simulink model "sampleModel1862"  (R2023a)
settings: Solver=VariableStepAuto  StartTime=0.0  StopTime=10.0  RelTol=1e-3
libraries: hdlsllib x1, simulink x1
settings Model: Creator=user1  LastModifiedBy=user1

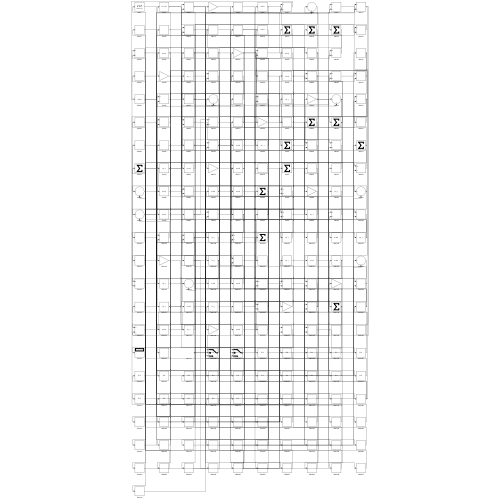
[thumbnail: Simulink's stored preview of the top-level diagram]
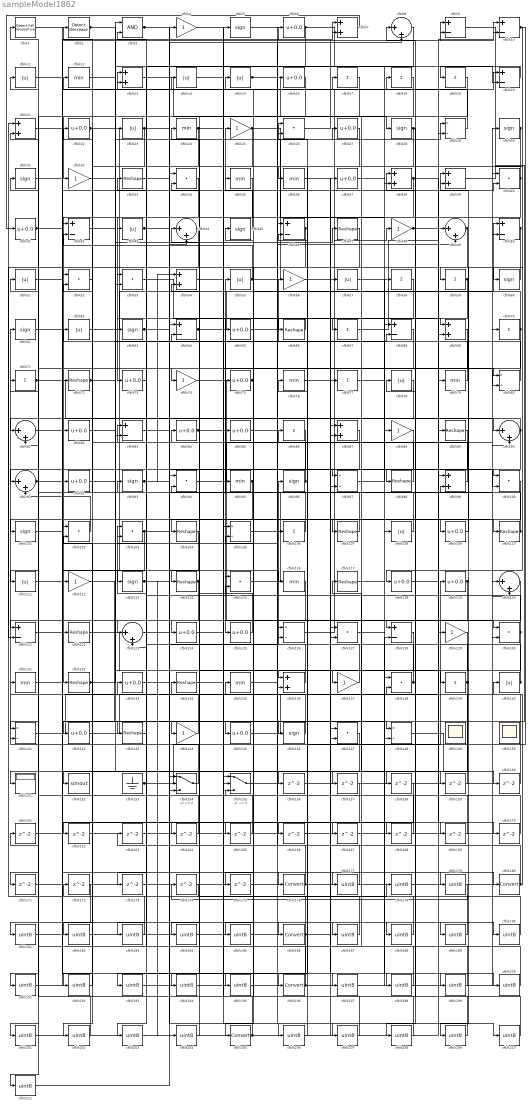
== system sampleModel1862 ==
  cfblk1 : hdlsllib/Logic and Bit Operations/Detect Fall Nonpositive  vinit=0  OutDataTypeStr=boolean
  cfblk{9..10,20,42,46,50,64,68,83,121,128} (11 alike) : Sum  Inputs=+-
  cfblk{26,34,40,52..53,94,100,102..103,115,127,130,138,147} (14 alike) : DotProduct  OutDataTypeStr=Inherit: Inherit via internal rule
  cfblk{5,28,30..31,45,60..61,63,93,96,101,113,146} (13 alike) : Signum
  cfblk{33,47,66,72,89,98,104,107,110,114,117,122,132,134,143} (15 alike) : Reshape
  cfblk{29,80,97,105,126,141,148} (7 alike) : Product  Inputs=*/  RndMeth=Zero  SaturateOnIntegerOverflow=on
  cfblk{17..19,58..59,67,70..71,77,86,106,139} (12 alike) : Sum  Inputs=+
  cfblk{11,14..15,23,43,51,55,57,62,78,108,111,140} (13 alike) : Abs  SaturateOnIntegerOverflow=off
  cfblk{6,16,22,27,37,41,65,73,75,82,84..85,92,109,118..119,124..125,133,142,145} (21 alike) : Bias  Bias=0.0  SaturateOnIntegerOverflow=off
  cfblk{4,25,32,48,56,74,88,112,129,137,144} (11 alike) : Gain
  cfblk{12,24,35..36,76,79,95,116,131,135} (10 alike) : MinMax
  cfblk{8,44,49,81,90..91,120,123} (8 alike) : Sum  Inputs=|++
  cfblk{7,13,21,38..39,54,69,87,99,136} (10 alike) : Sum
  cfblk149 : Scope
      settings: Floating=on
  cfblk150 : Scope
      settings: Floating=on
  cfblk151 : Display
  cfblk152 : ToWorkspace  VariableName=simout  SaveFormat=Timeseries  SampleTime=-1
  cfblk153 : Ground
  cfblk154 : Switch  SaturateOnIntegerOverflow=off  InputSameDT=off
  cfblk155 : Switch  SaturateOnIntegerOverflow=off  InputSameDT=off
  cfblk{156..175} (20 alike) : Delay  SampleTime=1
  cfblk{176,180,186,196,205} (5 alike) : DataTypeConversion  SaturateOnIntegerOverflow=off  RndMeth=Floor
  cfblk{177..179,181..185,187..195,197..204,206..211} (31 alike) : DataTypeConversion  OutDataTypeStr=uint8  SaturateOnIntegerOverflow=off  RndMeth=Floor
  cfblk2 : simulink/Logic and Bit Operations/Detect Decrease  vinit=0.0  OutDataTypeStr=boolean
      settings: LibrarySourceBlock=|
      | hdlsllib/Logic and Bit
      | Operations/Detect
      | Decrease
  cfblk3 : Logic  AllPortsSameDT=off  OutDataTypeStr=boolean
  wires:
  cfblk99/1 -> cfblk55/1
  cfblk44/1 -> cfblk132/1
  cfblk33/1 -> cfblk176/1
  cfblk113/1 -> cfblk204/1, cfblk206/1
  cfblk56/1 -> cfblk18/1
  cfblk22/1 -> cfblk114/1, cfblk82/1
  cfblk109/1 -> cfblk13/1
  cfblk38/1 -> cfblk73/1, cfblk170/1
  cfblk40/1 -> cfblk92/1, cfblk36/1
  cfblk55/1 -> cfblk29/1, cfblk42/2
  cfblk64/1 -> cfblk50/1, cfblk80/2
  cfblk85/1 -> cfblk130/1
  cfblk140/1 -> cfblk103/1, cfblk115/2
  cfblk46/1 -> cfblk104/1, cfblk65/1
  cfblk39/1 -> cfblk118/1
  cfblk126/1 -> cfblk48/1
  cfblk71/1 -> cfblk90/1, cfblk113/1
  cfblk60/1 -> cfblk59/1
  cfblk6/1 -> cfblk53/1, cfblk38/2
  cfblk154/1 -> cfblk61/1
  cfblk110/1 -> cfblk12/1, cfblk26/1
  cfblk96/1 -> cfblk91/1, cfblk52/2
  cfblk50/1 -> cfblk74/1, cfblk109/1
  cfblk112/1 -> cfblk144/1
  cfblk129/1 -> cfblk196/1
  cfblk70/1 -> cfblk39/2, cfblk181/1
  cfblk15/1 -> cfblk28/1, cfblk187/1
  cfblk63/1 -> cfblk9/1, cfblk87/2
  cfblk17/1 -> cfblk124/1
  cfblk80/1 -> cfblk56/1
  cfblk146/1 -> cfblk134/1
  cfblk9/1 -> cfblk148/1
  cfblk88/1 -> cfblk111/1
  cfblk62/1 -> cfblk16/1
  cfblk10/1 -> cfblk136/1, cfblk60/1
  cfblk108/1 -> cfblk15/1
  cfblk35/1 -> cfblk43/1
  cfblk20/1 -> cfblk19/1
  cfblk18/1 -> cfblk32/1
  cfblk45/1 -> cfblk25/1
  cfblk122/1 -> cfblk136/2
  cfblk91/1 -> cfblk148/2, cfblk159/1
  cfblk7/1 -> cfblk41/1
  cfblk145/1 -> cfblk89/1
  cfblk86/1 -> cfblk205/1
  cfblk29/1 -> cfblk2/1
  cfblk68/1 -> cfblk152/1
  cfblk74/1 -> cfblk128/1
  cfblk143/1 -> cfblk93/1
  cfblk98/1 -> cfblk24/1
  cfblk58/1 -> cfblk66/1
  cfblk138/1 -> cfblk83/1, cfblk38/1
  cfblk153/1 -> cfblk119/1, cfblk126/2
  cfblk84/1 -> cfblk64/2, cfblk20/1
  cfblk141/1 -> cfblk133/1
  cfblk144/1 -> cfblk11/1
  cfblk48/1 -> cfblk49/1, cfblk100/2
  cfblk82/1 -> cfblk3/1
  cfblk92/1 -> cfblk23/1
  cfblk53/1 -> cfblk69/1
  cfblk155/1 -> cfblk46/1
  cfblk135/1 -> cfblk49/2
  cfblk52/1 -> cfblk22/1
  cfblk87/1 -> cfblk151/1
  cfblk59/1 -> cfblk125/1, cfblk39/1
  cfblk95/1 -> cfblk141/1, cfblk162/1
  cfblk57/1 -> cfblk88/1
  cfblk137/1 -> cfblk35/1
  cfblk123/1 -> cfblk17/1
  cfblk42/1 -> cfblk27/1
  cfblk107/1 -> cfblk75/1
  cfblk67/1 -> cfblk10/1
  cfblk134/1 -> cfblk85/1
  cfblk94/1 -> cfblk70/1
  cfblk3/1 -> cfblk44/2, cfblk167/1
  cfblk83/1 -> cfblk155/2
  cfblk130/1 -> cfblk13/2, cfblk185/1
  cfblk125/1 -> cfblk44/1
  cfblk65/1 -> cfblk7/1
  cfblk24/1 -> cfblk122/1, cfblk80/1
  cfblk124/1 -> cfblk5/1
  cfblk136/1 -> cfblk96/1
  cfblk102/1 -> cfblk91/2
  cfblk106/1 -> cfblk71/1
  cfblk97/1 -> cfblk58/1
  cfblk100/1 -> cfblk123/1
  cfblk43/1 -> cfblk100/1, cfblk98/1
  cfblk132/1 -> cfblk139/1, cfblk68/2
  cfblk72/1 -> cfblk47/1, cfblk7/2
  cfblk36/1 -> cfblk57/1
  cfblk16/1 -> cfblk101/1
  cfblk79/1 -> cfblk62/1
  cfblk14/1 -> cfblk137/1
  cfblk28/1 -> cfblk158/1, cfblk184/1
  cfblk131/1 -> cfblk40/2
  cfblk127/1 -> cfblk180/1
  cfblk103/1 -> cfblk99/2, cfblk8/2, cfblk112/1
  cfblk115/1 -> cfblk90/2
  cfblk27/1 -> cfblk146/1
  cfblk32/1 -> cfblk116/1
  cfblk47/1 -> cfblk95/1
  cfblk75/1 -> cfblk45/1, cfblk175/1
  cfblk69/1 -> cfblk121/1
  cfblk114/1 -> cfblk171/1, cfblk192/1
  cfblk13/1 -> cfblk108/1
  cfblk119/1 -> cfblk143/1, cfblk208/1
  cfblk90/1 -> cfblk81/1, cfblk209/1
  cfblk12/1 -> cfblk53/2
  cfblk23/1 -> cfblk72/1, cfblk115/1, cfblk110/1
  cfblk93/1 -> cfblk145/1, cfblk54/1
  cfblk41/1 -> cfblk9/2, cfblk6/1
  cfblk104/1 -> cfblk154/2
  cfblk30/1 -> cfblk107/1, cfblk67/1
  cfblk49/1 -> cfblk121/2, cfblk97/1
  cfblk121/1 -> cfblk106/1
  cfblk73/1 -> cfblk3/2
  cfblk78/1 -> cfblk154/3
  cfblk2/1 -> cfblk20/2, cfblk156/1
  cfblk26/1 -> cfblk10/2
  cfblk142/1 -> cfblk87/1
  cfblk25/1 -> cfblk68/1, cfblk83/2, cfblk97/2
  cfblk66/1 -> cfblk63/1
  cfblk118/1 -> cfblk79/1
  cfblk8/1 -> cfblk123/2
  cfblk31/1 -> cfblk186/1
  cfblk101/1 -> cfblk14/1
  cfblk139/1 -> cfblk142/1, cfblk8/1, cfblk201/1
  cfblk156/1 -> cfblk50/2
  cfblk19/1 -> cfblk157/1
  cfblk159/1 -> cfblk99/1
  cfblk148/1 -> cfblk160/1
  cfblk160/1 -> cfblk46/2
  cfblk161/1 -> cfblk42/1
  cfblk162/1 -> cfblk155/1
  cfblk163/1 -> cfblk130/2
  cfblk81/1 -> cfblk164/1
  cfblk164/1 -> cfblk64/1
  cfblk51/1 -> cfblk165/1
  cfblk165/1 -> cfblk154/1
  cfblk54/1 -> cfblk166/1
  cfblk166/1 -> cfblk69/2
  cfblk167/1 -> cfblk40/1
  cfblk5/1 -> cfblk168/1
  cfblk168/1 -> cfblk1/1
  cfblk117/1 -> cfblk169/1
  cfblk169/1 -> cfblk94/1
  cfblk170/1 -> cfblk155/3
  cfblk171/1 -> cfblk128/2
  cfblk116/1 -> cfblk173/1
  cfblk173/1 -> cfblk103/2
  cfblk175/1 -> cfblk30/1
  cfblk176/1 -> cfblk135/1, cfblk84/1
  cfblk1/1 -> cfblk177/1
  cfblk177/1 -> cfblk33/1
  cfblk174/1 -> cfblk178/1
  cfblk178/1 -> cfblk138/2
  cfblk11/1 -> cfblk179/1
  cfblk179/1 -> cfblk174/1
  cfblk180/1 -> cfblk26/2, cfblk126/1, cfblk140/1
  cfblk181/1 -> cfblk127/1
  cfblk157/1 -> cfblk182/1
  cfblk182/1 -> cfblk127/2
  cfblk147/1 -> cfblk183/1
  cfblk183/1 -> cfblk102/2
  cfblk184/1 -> cfblk147/1
  cfblk185/1 -> cfblk147/2
  cfblk186/1 -> cfblk131/1, cfblk203/1
  cfblk187/1 -> cfblk31/1
  cfblk21/1 -> cfblk188/1
  cfblk188/1 -> cfblk102/1
  cfblk37/1 -> cfblk189/1
  cfblk189/1 -> cfblk21/1
  cfblk111/1 -> cfblk190/1
  cfblk190/1 -> cfblk21/2
  cfblk172/1 -> cfblk191/1
  cfblk191/1 -> cfblk52/1
  cfblk192/1 -> cfblk172/1
  cfblk120/1 -> cfblk193/1
  cfblk193/1 -> cfblk138/1
  cfblk128/1 -> cfblk194/1
  cfblk194/1 -> cfblk120/1
  cfblk158/1 -> cfblk195/1
  cfblk195/1 -> cfblk120/2
  cfblk196/1 -> cfblk163/1, cfblk81/2
  cfblk133/1 -> cfblk197/1
  cfblk197/1 -> cfblk129/1
  cfblk76/1 -> cfblk198/1
  cfblk198/1 -> cfblk94/2
  cfblk61/1 -> cfblk199/1
  cfblk199/1 -> cfblk76/1
  cfblk77/1 -> cfblk200/1
  cfblk200/1 -> cfblk117/1
  cfblk201/1 -> cfblk77/1
  cfblk34/1 -> cfblk202/1
  cfblk202/1 -> cfblk161/1
  cfblk203/1 -> cfblk34/1
  cfblk204/1 -> cfblk34/2
  cfblk205/1 -> cfblk54/2, cfblk141/2, cfblk37/1, cfblk29/2
  cfblk206/1 -> cfblk86/1
  cfblk105/1 -> cfblk207/1
  cfblk207/1 -> cfblk51/1
  cfblk208/1 -> cfblk105/1
  cfblk209/1 -> cfblk105/2
  cfblk4/1 -> cfblk210/1
  cfblk210/1 -> cfblk78/1
  cfblk89/1 -> cfblk211/1
  cfblk211/1 -> cfblk4/1
